simulink model "tau"  (R2023a)
settings: Solver=VariableStepAuto  StartTime=0.0  StopTime=2  RelTol=1e-3
libraries: simulink x7
settings Model: Creator=User  LastModifiedBy=User

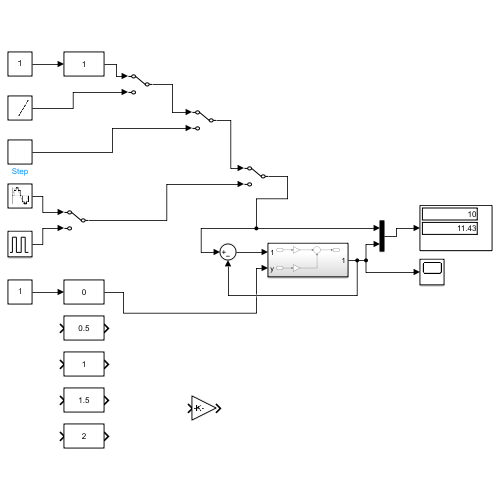
[thumbnail: Simulink's stored preview of the top-level diagram]
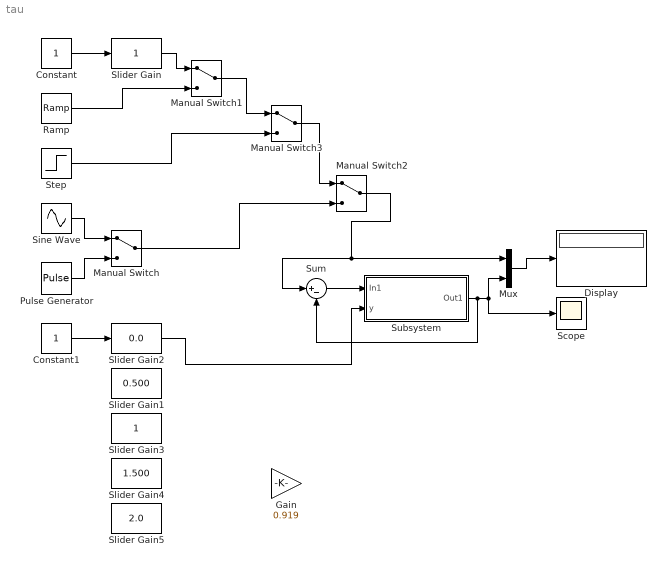
== system tau ==
  Constant : Constant
  Constant1 : Constant
  Display : Display
  Gain : Gain  Gain=0.919
  Manual Switch{,1..3} (4 alike) : ManualSwitch
  Mux : Mux  Inputs=2
  Pulse Generator : DiscretePulseGenerator  PulseType=Time based  Period=0.1  PulseWidth=50
  Ramp : simulink/Sources/Ramp  slope=10  start=0  InitialOutput=0
  Scope : Scope
  Sine Wave : Sin  Frequency=10*2*pi  SampleTime=0.0001
  Slider Gain : simulink/Math Operations/Slider Gain  gain=1  low=0  high=2
  Slider Gain1 : simulink/Math Operations/Slider Gain  gain=0.500  low=0  high=2
  Slider Gain2 : simulink/Math Operations/Slider Gain  gain=0.0  low=0  high=2
  Slider Gain3 : simulink/Math Operations/Slider Gain  gain=1  low=0  high=2
  Slider Gain4 : simulink/Math Operations/Slider Gain  gain=1.500  low=0  high=2
  Slider Gain5 : simulink/Math Operations/Slider Gain  gain=2.0  low=0  high=2
  Step : Step  Time=0.1  SampleTime=0
  Subsystem : Subsystem
  Sum : Sum  Inputs=|+-
  wires:
  Sine Wave/1 -> Manual Switch/1
  Pulse Generator/1 -> Manual Switch/2
  Constant/1 -> Slider Gain/1
  Constant1/1 -> Slider Gain2/1
  Slider Gain/1 -> Manual Switch1/1
  Ramp/1 -> Manual Switch1/2
  Manual Switch1/1 -> Manual Switch3/1
  Step/1 -> Manual Switch3/2
  Manual Switch3/1 -> Manual Switch2/1
  Manual Switch/1 -> Manual Switch2/2
  Manual Switch2/1 -> Mux/1, Sum/1
  Slider Gain2/1 -> Subsystem/2(y)
  Subsystem/1(Out1) -> Sum/2, Mux/2, Scope/1
  Mux/1 -> Display/1
  Sum/1 -> Subsystem/1(In1)

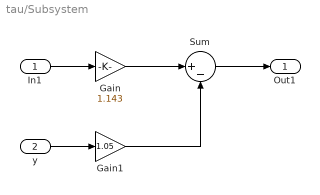
== system tau/Subsystem ==
  In1 : Inport
  y : Inport  Port=2
  Gain : Gain  Gain=1.143
  Gain1 : Gain  Gain=1.05
  Sum : Sum  Inputs=|+-
  Out1 : Outport
  wires:
  In1/1 -> Gain/1
  y/1 -> Gain1/1
  Gain1/1 -> Sum/2
  Gain/1 -> Sum/1
  Sum/1 -> Out1/1
